simulink model "Practica3_Simulink"  (R2024a)
settings: Solver=VariableStepAuto  StartTime=0.0  StopTime=10.0  RelTol=1e-3
InitFcn:
  | m1 = 290;
  | b1 = 1000;
  | m2 = 59;
  | k1 = 16182;
  | f = 0;
  | k2 = 19000;
settings Model: Creator=Manuel  LastModifiedBy=Manuel

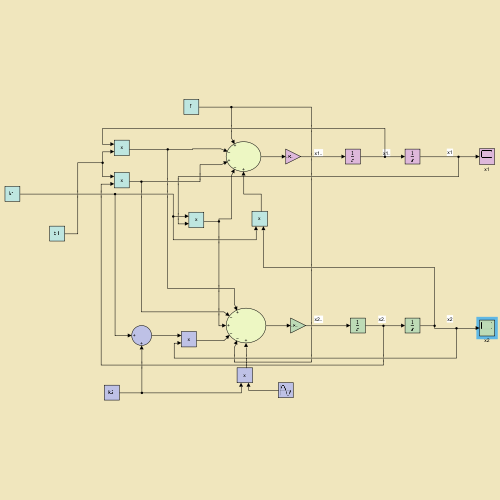
[thumbnail: Simulink's stored preview of the top-level diagram]
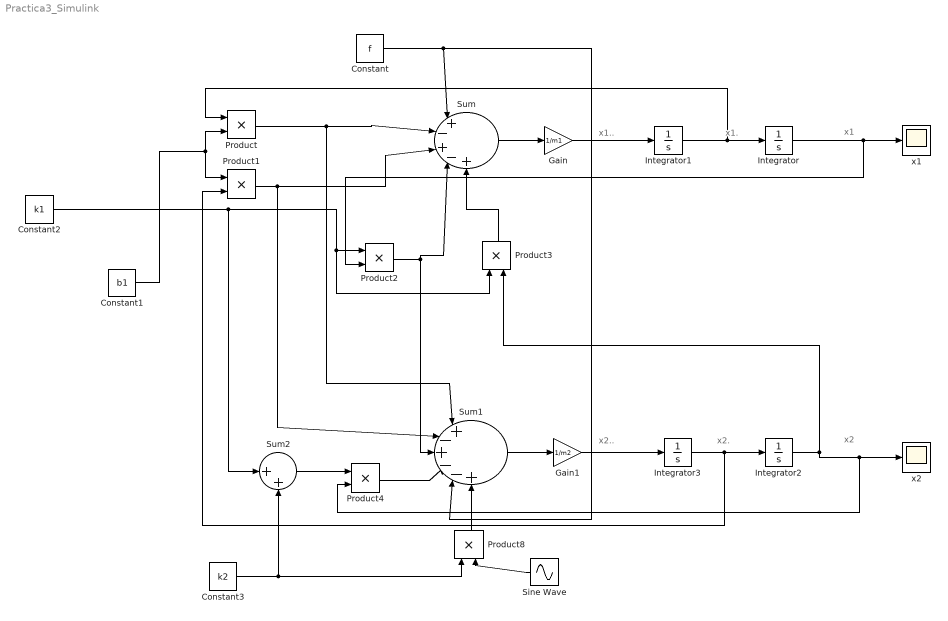
== system Practica3_Simulink ==
  note: x1.
  note: x2
  note: x1
  note: x1..
  note: x2..
  note: x2.
  Constant : Constant  Value=f
  Constant1 : Constant  Value=b1
  Constant2 : Constant  Value=k1
  Constant3 : Constant  Value=k2
  Gain : Gain  Gain=1/m1
  Gain1 : Gain  Gain=1/m2
  Integrator{,1..3} (4 alike) : Integrator
  Product{,1..4,8} (6 alike) : Product
  Sine Wave : Sin  Amplitude=.05  Frequency=.5*pi  SampleTime=0
  Sum : Sum  Inputs=|+-+-+
  Sum1 : Sum  Inputs=|+-+--+
  Sum2 : Sum  Inputs=|++
  x1 : Scope
  x2 : Scope
  wires:
  Product8/1 -> Sum1/6
  Sine Wave/1 -> Product8/2
  Product3/1 -> Sum/5
  Product1/1 -> Sum/3, Sum1/2
  Gain1/1 -> Integrator3/1
  Sum/1 -> Gain/1
  Integrator2/1 -> Product3/2, Product4/2, x2/1
  Integrator1/1 -> Product/1, Integrator/1
  Constant1/1 -> Product1/1, Product/2
  Gain/1 -> Integrator1/1
  Sum1/1 -> Gain1/1
  Integrator/1 -> Product2/2, x1/1
  Product2/1 -> Sum1/3, Sum/4
  Constant2/1 -> Sum2/1, Product3/1, Product2/1
  Constant/1 -> Sum1/5, Sum/1
  Product/1 -> Sum/2, Sum1/1
  Integrator3/1 -> Product1/2, Integrator2/1
  Sum2/1 -> Product4/1
  Constant3/1 -> Product8/1, Sum2/2
  Product4/1 -> Sum1/4
